simulink model "feedbackControl"  (R2020a)
settings: Solver=VariableStepAuto  StartTime=0.0  StopTime=10.0  MaxStep=0.01  RelTol=1e-3
values from neighbouring files (symbols this model uses):
  L = lqr(A, B, Q, R)    [code.m]    (also in main.m = lqrL)
  L_r = pinv(C*inv(-A + B*L)*B)    [code.m]    (also in main.m = lqrL_r)
libraries: helperLibrary x1
settings Model: Creator=danth  LastModifiedBy=danth

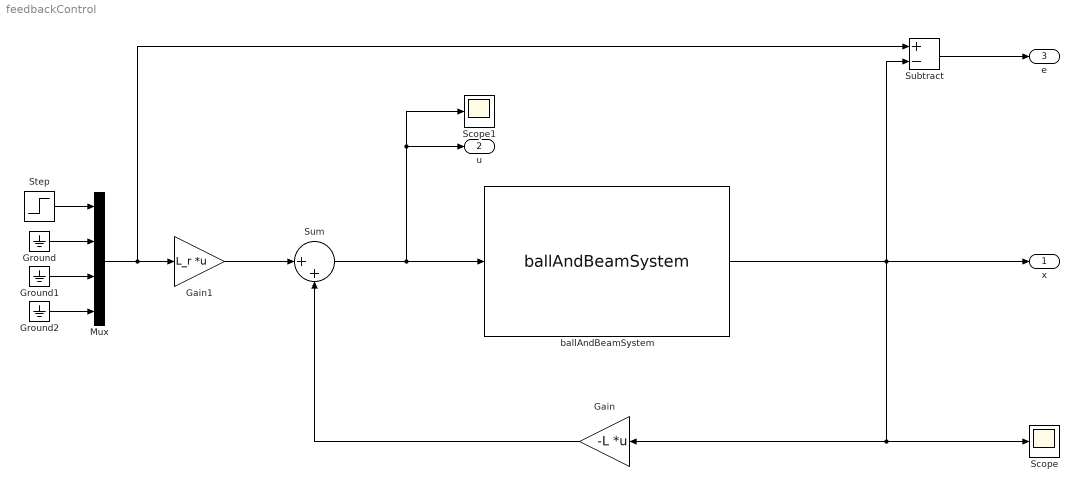
== system feedbackControl ==
  Gain : Gain  Gain=-L  Multiplication=Matrix(K*u)
  Gain1 : Gain  Gain=L_r  Multiplication=Matrix(K*u)
  Ground : Ground
  Ground1 : Ground
  Ground2 : Ground
  Mux : Mux
  Scope : Scope
  Scope1 : Scope
  Step : Step  Time=0  After=0  SampleTime=0
  Subtract : Sum  Inputs=+-
  Sum : Sum  Inputs=|++
  ballAndBeamSystem : helperLibrary/ballAndBeamSystem  SystemSampleTime=-1  Latency=0  AutoFrameSizeCalculation=off
  x : Outport
  u : Outport  Port=2
  e : Outport  Port=3
  wires:
  ballAndBeamSystem/1 -> Gain/1, Scope/1, Subtract/2, x/1
  Sum/1 -> u/1, Scope1/1, ballAndBeamSystem/1
  Gain/1 -> Sum/2
  Gain1/1 -> Sum/1
  Mux/1 -> Subtract/1, Gain1/1
  Step/1 -> Mux/1
  Ground/1 -> Mux/2
  Ground1/1 -> Mux/3
  Ground2/1 -> Mux/4
  Subtract/1 -> e/1
